simulink model "Lab11"  (R2025b)
settings: Solver=VariableStepAuto  StartTime=0.0  StopTime=100  RelTol=1e-3
libraries: simulink x2
settings Model: Creator=rares  LastModifiedBy=rares

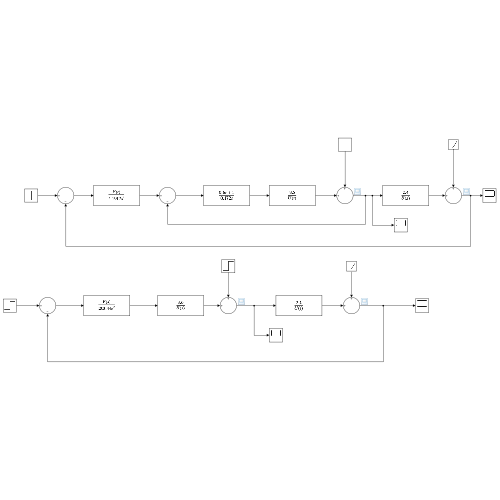
[thumbnail: Simulink's stored preview of the top-level diagram]
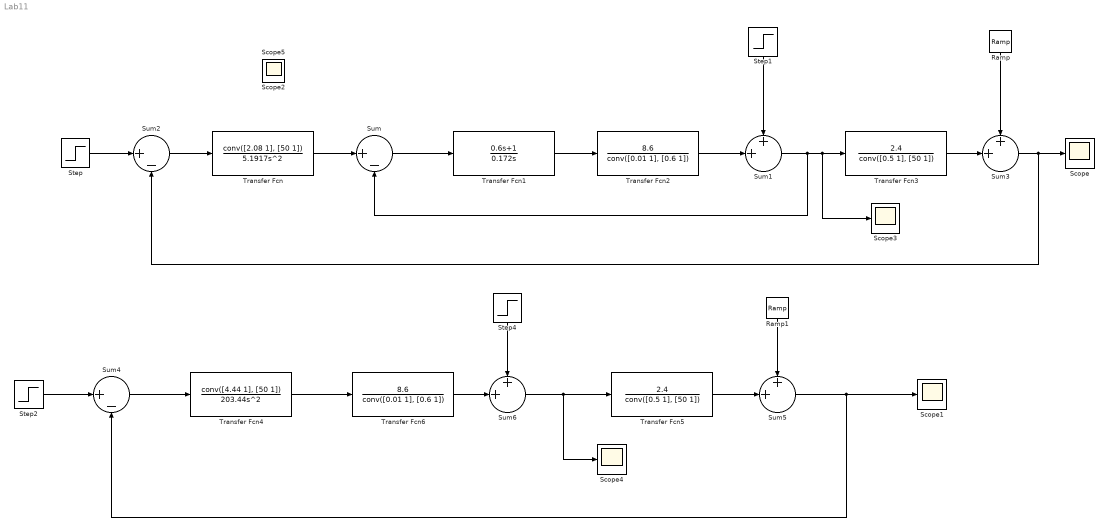
== system Lab11 ==
  Ramp : simulink/Sources/Ramp  slope=1  start=40  InitialOutput=0
  Ramp1 : simulink/Sources/Ramp  slope=1  start=40  InitialOutput=0
  Scope{,1..5} (6 alike) : Scope
      Scope settings: ActiveDisplayYMinimum=-1  ActiveDisplayYMaximum=1
      Scope1 settings: ActiveDisplayYMinimum=-1  ActiveDisplayYMaximum=1
      Scope3 settings: ActiveDisplayYMinimum=-1  ActiveDisplayYMaximum=1  DataLoggingVariableName=ScopeData3
      Scope4 settings: ActiveDisplayYMinimum=-1  ActiveDisplayYMaximum=1  DataLoggingVariableName=ScopeData4
      Scope2 settings: ActiveDisplayYMinimum=-0.21984289061030871  ActiveDisplayYMaximum=2.1812926534764463  DataLoggingVariableName=ScopeData2
      Scope5 settings: ActiveDisplayYMinimum=-1.8808066197915667  ActiveDisplayYMaximum=1.7137045904887347  DataLoggingVariableName=ScopeData5
  Step : Step  SampleTime=0
  Step1 : Step  Time=20  SampleTime=0
  Step2 : Step  SampleTime=0
  Step4 : Step  Time=20  SampleTime=0
  Sum : Sum  Inputs=|+-
  Sum{1,3,5..6} (4 alike) : Sum  Inputs=++|
  Sum2 : Sum  Inputs=|+-
  Sum4 : Sum  Inputs=|+-
  Transfer Fcn : TransferFcn  Numerator=conv([2.08 1], [50 1])  Denominator=[5.1917 0 0]
  Transfer Fcn1 : TransferFcn  Numerator=[0.6 1]  Denominator=[0.172 0]
  Transfer Fcn2 : TransferFcn  Numerator=8.6  Denominator=conv([0.01 1], [0.6 1])
  Transfer Fcn3 : TransferFcn  Numerator=2.4  Denominator=conv([0.5 1], [50 1])
  Transfer Fcn4 : TransferFcn  Numerator=conv([4.44 1], [50 1])  Denominator=[203.44 0 0]
  Transfer Fcn5 : TransferFcn  Numerator=2.4  Denominator=conv([0.5 1], [50 1])
  Transfer Fcn6 : TransferFcn  Numerator=8.6  Denominator=conv([0.01 1], [0.6 1])
  wires:
  Sum2/1 -> Transfer Fcn/1
  Transfer Fcn/1 -> Sum/1
  Sum/1 -> Transfer Fcn1/1
  Transfer Fcn1/1 -> Transfer Fcn2/1
  Transfer Fcn2/1 -> Sum1/2
  Sum1/1 -> Sum/2, Scope3/1, Transfer Fcn3/1
  Transfer Fcn3/1 -> Sum3/2
  Step/1 -> Sum2/1
  Step1/1 -> Sum1/1
  Ramp/1 -> Sum3/1
  Sum3/1 -> Sum2/2, Scope/1
  Sum4/1 -> Transfer Fcn4/1
  Transfer Fcn4/1 -> Transfer Fcn6/1
  Step2/1 -> Sum4/1
  Ramp1/1 -> Sum5/1
  Transfer Fcn6/1 -> Sum6/2
  Sum6/1 -> Scope4/1, Transfer Fcn5/1
  Step4/1 -> Sum6/1
  Transfer Fcn5/1 -> Sum5/2
  Sum5/1 -> Sum4/2, Scope1/1
